simulink model "L6"  (R2019b)
settings: Solver=VariableStepAuto  StartTime=0.0  StopTime=50  RelTol=1e-3
InitFcn:
  | %% Параметры механизма
  | m = [1 1];      % масса звеньев
  | l = [1 1];      % длина звеньев
  | lc = [.5 .5];   % расст от СК звена до центра масс звена
  | I = [1 1];      % моменты инерции звеньев
  | Jm = [0 0];     % момент инерции редукторов?
  | r = [1 1];      % передаточные числа редукторов
  | D = [.1 .1];    % агрегированные коэффициенты демпфирования
  | 
  | g = 9.81;       % ускорение свободного падения
  | 
  | 
  | global rho;
  | rho = [
  |     m(1)*lc(1)^2 + m(2)*l(1)^2 + 2*m(2)*l(1)*lc(2)^2 + I(1),... % rho_1
  |     m(2)*lc(2)^2 + I(2),...                                     % rho_2
  |     m(2)*l(1)*lc(2),...                                         % rho_3
  |     r(1)^2*Jm(1),...                                            % rho_4
  |     r(2)^2*Jm(2),...                                            % rho_5
  |     (m(1)*lc(1) + m(2)*l(1))*g,...                              % rho_6
  |     m(2)*lc(2)*g,...                                            % rho_7
  |     m(2)*lc(2),...                                              % rho_8
  |     r(1)^2*D(1),...                                             % rho_9
  |     r(2)^2*D(2)                                                 % rho_10
  |     ];
  | 
  | 
  | q_ref = [1 2];
  | c2 = cos(q_ref(2));
  | 
  | % матрица номинального момента инерции манипулятора
  | M0 = [
  |     rho(1) + rho(2) + 2*rho(3)*c2 + rho(4), rho(2) + rho(3)*c2;
  |     rho(2) + rho(3)*c2, rho(2) + rho(5);
  |     ];
  | 
  | % матрица вязкого трения
  | Friction = [
  |     rho(9) 0;
  |     0 rho(10)
  |     ];
  | 
  | %% Параметры генераторов
  | % Задающий блок
  | A_ref = [1 1];      % амплитуды
  | psi_ref = [0 0];    % фазы
  | omega_ref = [1 2];  % частоты
  | 
  | w_ref_0 = [
  |     A_ref(1)*sin(psi_ref(1)),...
  |     omega_ref(1)*A_ref(1)*cos(psi_ref(1)),...
  |     A_ref(2)*sin(psi_ref(2)),...
  |     omega_ref(2)*A_ref(2)*cos(psi_ref(2))
  |     ]';
  | 
  | Sref1 = [
  |     0 1;
  |     -omega_ref(1)^2 0
  |     ];
  | Sref2 = [
  |     0 1;
  |     -omega_ref(2)^2 0
  |     ];
  | 
  | Sref = blkdiag(Sref1, Sref2);
  | 
  | H_ref_p1 = [1 0];
  | H_ref_p2 = [1 0];
  | H_ref_p = blkdiag(H_ref_p1, H_ref_p2);
  | 
  | H_ref_v1 = [0 1];
  | H_ref_v2 = [0 1];
  | H_ref_v = blkdiag(H_ref_v1, H_ref_v2);
  | 
  | H_ref_a1 = [-omega_ref(1)^2 0];
  | H_ref_a2 = [-omega_ref(2)^2 0];
  | H_ref_a = blkdiag(H_ref_a1, H_ref_a2);
  | 
  | % Возмущающий блок
  | A_dist = [30 40];       % амплитуды
  | C_dist = [5 6];         % свободный член
  | psi_dist = [7 8];       % фазы
  | omega_dist = [1 2];     % частоты
  | 
  | w_dist_0 = [
  |     C_dist(1);
  |     A_dist(1)*sin(psi_dist(1));
  |     omega_dist(1)*A_dist(1)*cos(psi_dist(1));
  |     C_dist(2);
  |     A_dist(2)*sin(psi_dist(2));
  |     omega_dist(2)*A_dist(2)*cos(psi_dist(2))
  |     ];
  | 
  | Sdist1 = [
  |     0 0 0
  |     0 0 1;
  |     0 -omega_dist(1)^2 0
  |     ];
  | Sdist2 = [
  |     0 0 0
  |     0 0 1;
  |     0 -omega_dist(2)^2 0
  |     ];
  | 
  | Sdist = blkdiag(Sdist1, Sdist2);
  | 
  | H_dist_1 = [1 1 0];
  | H_dist_2 = [1 1 0];
  | H_dist = blkdiag(H_dist_1, H_dist_2);
  | 
  | f = [1 3 3];
  | F_1 =[
  |     zeros(2, 1) eye(2);
  |     -f
  |     ];
  | F_2 =[
  |     zeros(2, 1) eye(2);
  |     -f
  |     ];
  | F = blkdiag(F_1, F_2);
  | 
  | G_1 = [0 0 1]';
  | G_2 = [0 0 1]';
  | G = blkdiag(G_1, G_2);
  | 
  | Gamma_1 = f - [0 omega_dist(1)^2 0];
  | Gamma_2 = f - [0 omega_dist(2)^2 0];
  | Gamma = blkdiag(Gamma_1, Gamma_2);
  | %% Параметры регулятора
  | kappa = 1000;
  | 
  | K =[
  |     1 0 1 0;
  |     0 1 0 1
  |     ];
  | 
  | N = inf;
  | 
  | A0 = [
  |     30 3;
  |     3 30
  |     ];
  | A1 = [
  |     30 3;
  |     3 30
  |     ];
  | A2 = [
  |     10 1;
  |     1 10
  |     ];
  | 
  | A = [
  |     -A2 eye(size(A2)) zeros(size(A2));
  |     -A1 zeros(size(A1)) eye(size(A1));
  |     -A0 zeros(size(A0)) zeros(size(A0));
  |     ];
  | % остальные матрицы зависят от q и объявлены функциями
settings Model: Creator=bedla  LastModifiedBy=bedla

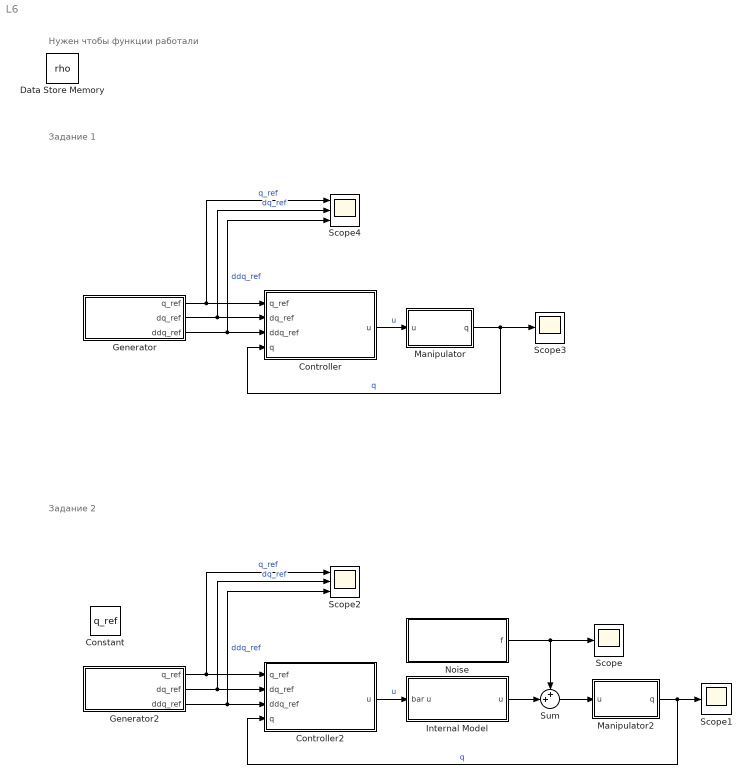
== system L6 ==
  note: Задание 1
  note: Нужен чтобы функции работали
  note: Задание 2
  Constant : Constant  Value=q_ref
  Controller : Subsystem
  Controller2 : Subsystem
  Data Store Memory : DataStoreMemory  DataStoreName=rho  ReadBeforeWriteMsg=warning  WriteAfterWriteMsg=warning  WriteAfterReadMsg=warning  InitialValue=rho  ShowAdditionalParam=off  OutDataTypeStr=double
  Generator : Subsystem
  Generator2 : Subsystem
  Internal Model : Subsystem
  Manipulator : Subsystem
  Manipulator2 : Subsystem
  Noise : Subsystem
  Scope : Scope
  Scope1 : Scope
  Scope2 : Scope  NumInputPorts=3
  Scope3 : Scope
  Scope4 : Scope  NumInputPorts=3
  Sum : Sum  Inputs=++|
  wires:
  Generator/1(q_ref) -> Controller/1(q_ref), Scope4/1  "q_ref"
  Manipulator/1(q) -> Controller/4(q), Scope3/1  "q"
  Generator/3(ddq_ref) -> Controller/3(ddq_ref), Scope4/3  "ddq_ref"
  Controller/1(u) -> Manipulator/1(u)  "u"
  Generator/2(dq_ref) -> Controller/2(dq_ref), Scope4/2  "dq_ref"
  Generator2/2(dq_ref) -> Controller2/2(dq_ref), Scope2/2  "dq_ref"
  Generator2/3(ddq_ref) -> Controller2/3(ddq_ref), Scope2/3  "ddq_ref"
  Generator2/1(q_ref) -> Scope2/1, Controller2/1(q_ref)  "q_ref"
  Controller2/1(u) -> Internal Model/1(bar u)  "u"
  Manipulator2/1(q) -> Controller2/4(q), Scope1/1  "q"
  Sum/1 -> Manipulator2/1(u)
  Noise/1(f) -> Scope/1, Sum/1
  Internal Model/1(u) -> Sum/2

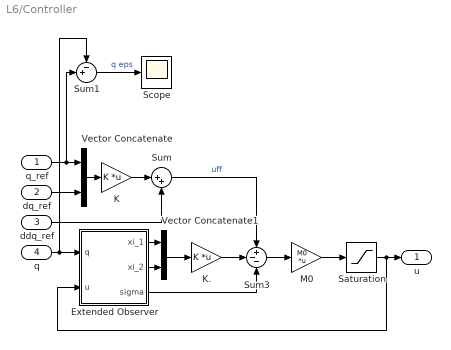
== system L6/Controller ==
  q_ref : Inport
  dq_ref : Inport  Port=2
  ddq_ref : Inport  Port=3
  q : Inport  Port=4
  Extended Observer : Subsystem
  K : Gain  Gain=K  Multiplication=Matrix(K*u) (u vector)
  K. : Gain  Gain=K  Multiplication=Matrix(K*u) (u vector)
  M0 : Gain  Gain=M0  Multiplication=Matrix(K*u) (u vector)
  Saturation : Saturate  UpperLimit=N  LowerLimit=-N
  Scope : Scope
  Sum : Sum  Inputs=|++
  Sum1 : Sum  Inputs=-+|
  Sum3 : Sum  Inputs=+--
  Vector Concatenate : Concatenate
  Vector Concatenate1 : Concatenate
  u : Outport
  wires:
  Saturation/1 -> Extended Observer/2(u), u/1
  dq_ref/1 -> Vector Concatenate/2
  q_ref/1 -> Sum1/2, Vector Concatenate/1
  Vector Concatenate/1 -> K/1
  K/1 -> Sum/1
  ddq_ref/1 -> Sum/2
  Sum3/1 -> M0/1
  Extended Observer/3(sigma) -> Sum3/3
  K./1 -> Sum3/2
  M0/1 -> Saturation/1
  Extended Observer/2(xi_2) -> Vector Concatenate1/2
  Sum/1 -> Sum3/1  "uff"
  q/1 -> Sum1/1, Extended Observer/1(q)
  Extended Observer/1(xi_1) -> Vector Concatenate1/1
  Vector Concatenate1/1 -> K./1
  Sum1/1 -> Scope/1  "q eps"

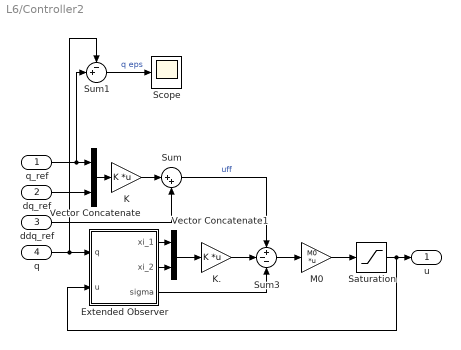
== system L6/Controller2 ==
  q_ref : Inport
  dq_ref : Inport  Port=2
  ddq_ref : Inport  Port=3
  q : Inport  Port=4
  Extended Observer : Subsystem
  K : Gain  Gain=K  Multiplication=Matrix(K*u) (u vector)
  K. : Gain  Gain=K  Multiplication=Matrix(K*u) (u vector)
  M0 : Gain  Gain=M0  Multiplication=Matrix(K*u) (u vector)
  Saturation : Saturate  UpperLimit=N  LowerLimit=-N
  Scope : Scope
  Sum : Sum  Inputs=|++
  Sum1 : Sum  Inputs=-+|
  Sum3 : Sum  Inputs=+--
  Vector Concatenate : Concatenate
  Vector Concatenate1 : Concatenate
  u : Outport
  wires:
  Saturation/1 -> Extended Observer/2(u), u/1
  dq_ref/1 -> Vector Concatenate/2
  q_ref/1 -> Sum1/2, Vector Concatenate/1
  Vector Concatenate/1 -> K/1
  K/1 -> Sum/1
  ddq_ref/1 -> Sum/2
  Sum3/1 -> M0/1
  Extended Observer/3(sigma) -> Sum3/3
  K./1 -> Sum3/2
  M0/1 -> Saturation/1
  Extended Observer/2(xi_2) -> Vector Concatenate1/2
  Sum/1 -> Sum3/1  "uff"
  q/1 -> Sum1/1, Extended Observer/1(q)
  Extended Observer/1(xi_1) -> Vector Concatenate1/1
  Vector Concatenate1/1 -> K./1
  Sum1/1 -> Scope/1  "q eps"

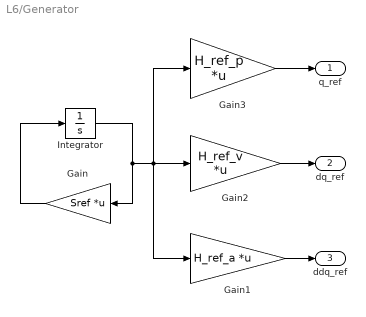
== system L6/Generator ==
  Gain : Gain  Gain=Sref  Multiplication=Matrix(K*u) (u vector)
  Gain1 : Gain  Gain=H_ref_a  Multiplication=Matrix(K*u) (u vector)
  Gain2 : Gain  Gain=H_ref_v  Multiplication=Matrix(K*u) (u vector)
  Gain3 : Gain  Gain=H_ref_p  Multiplication=Matrix(K*u) (u vector)
  Integrator : Integrator  InitialCondition=w_ref_0
  q_ref : Outport
  dq_ref : Outport  Port=2
  ddq_ref : Outport  Port=3
  wires:
  Gain/1 -> Integrator/1
  Integrator/1 -> Gain/1, Gain3/1, Gain2/1, Gain1/1
  Gain1/1 -> ddq_ref/1
  Gain2/1 -> dq_ref/1
  Gain3/1 -> q_ref/1

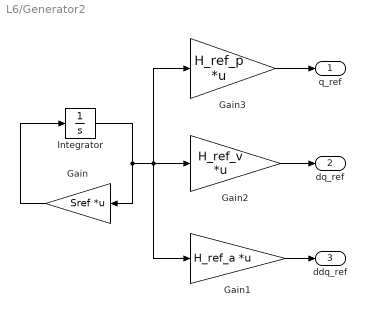
== system L6/Generator2 ==
  Gain : Gain  Gain=Sref  Multiplication=Matrix(K*u) (u vector)
  Gain1 : Gain  Gain=H_ref_a  Multiplication=Matrix(K*u) (u vector)
  Gain2 : Gain  Gain=H_ref_v  Multiplication=Matrix(K*u) (u vector)
  Gain3 : Gain  Gain=H_ref_p  Multiplication=Matrix(K*u) (u vector)
  Integrator : Integrator  InitialCondition=w_ref_0
  q_ref : Outport
  dq_ref : Outport  Port=2
  ddq_ref : Outport  Port=3
  wires:
  Gain/1 -> Integrator/1
  Integrator/1 -> Gain/1, Gain3/1, Gain2/1, Gain1/1
  Gain1/1 -> ddq_ref/1
  Gain2/1 -> dq_ref/1
  Gain3/1 -> q_ref/1

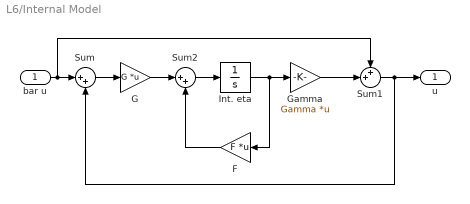
== system L6/Internal Model ==
  bar u : Inport
  F : Gain  Gain=F  Multiplication=Matrix(K*u)
  G : Gain  Gain=G  Multiplication=Matrix(K*u)
  Gamma : Gain  Gain=Gamma  Multiplication=Matrix(K*u)
  Int. eta : Integrator
  Sum : Sum  Inputs=|++
  Sum1 : Sum  Inputs=++|
  Sum2 : Sum  Inputs=|++
  u : Outport
  wires:
  bar u/1 -> Sum1/1, Sum/1
  Sum1/1 -> Sum/2, u/1
  Sum/1 -> G/1
  Gamma/1 -> Sum1/2
  Int. eta/1 -> F/1, Gamma/1
  G/1 -> Sum2/1
  Sum2/1 -> Int. eta/1
  F/1 -> Sum2/2

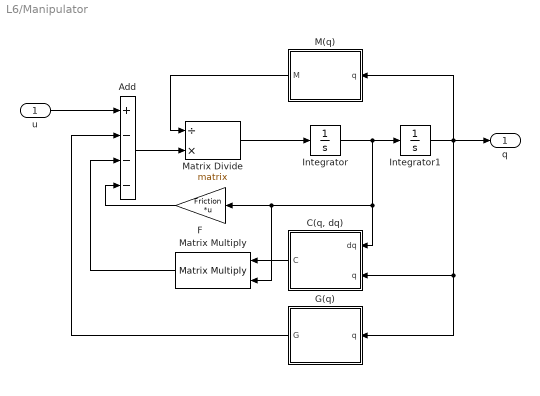
== system L6/Manipulator ==
  u : Inport
  Add : Sum  Inputs=+---
  "C(q, dq)" : MATLAB Function
  F : Gain  Gain=Friction  Multiplication=Matrix(K*u) (u vector)
  G(q) : MATLAB Function  TreatAsAtomicUnit=on
  Integrator : Integrator
  Integrator1 : Integrator
  M(q) : MATLAB Function  TreatAsAtomicUnit=on
  Matrix Divide : Product  Inputs=/*  Multiplication=Matrix(*)
  Matrix Multiply : Product  Multiplication=Matrix(*)
  q : Outport
  wires:
  Matrix Divide/1 -> Integrator/1
  Add/1 -> Matrix Divide/2
  Integrator/1 -> "C(q, dq)"/1(dq), Matrix Multiply/2, F/1, Integrator1/1
  Matrix Multiply/1 -> Add/3
  Integrator1/1 -> q/1, M(q)/1(q), G(q)/1(q), "C(q, dq)"/2(q)
  M(q)/1(M) -> Matrix Divide/1
  u/1 -> Add/1
  G(q)/1(G) -> Add/2
  "C(q, dq)"/1(C) -> Matrix Multiply/1
  F/1 -> Add/4

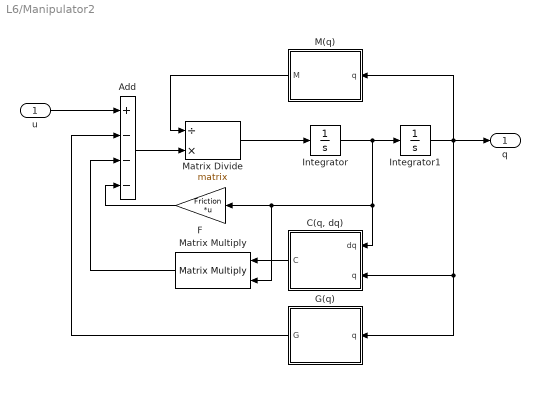
== system L6/Manipulator2 ==
  u : Inport
  Add : Sum  Inputs=+---
  "C(q, dq)" : MATLAB Function
  F : Gain  Gain=Friction  Multiplication=Matrix(K*u) (u vector)
  G(q) : MATLAB Function  TreatAsAtomicUnit=on
  Integrator : Integrator
  Integrator1 : Integrator
  M(q) : MATLAB Function  TreatAsAtomicUnit=on
  Matrix Divide : Product  Inputs=/*  Multiplication=Matrix(*)
  Matrix Multiply : Product  Multiplication=Matrix(*)
  q : Outport
  wires:
  Matrix Divide/1 -> Integrator/1
  Add/1 -> Matrix Divide/2
  Integrator/1 -> "C(q, dq)"/1(dq), Matrix Multiply/2, F/1, Integrator1/1
  Matrix Multiply/1 -> Add/3
  Integrator1/1 -> q/1, M(q)/1(q), G(q)/1(q), "C(q, dq)"/2(q)
  M(q)/1(M) -> Matrix Divide/1
  u/1 -> Add/1
  G(q)/1(G) -> Add/2
  "C(q, dq)"/1(C) -> Matrix Multiply/1
  F/1 -> Add/4

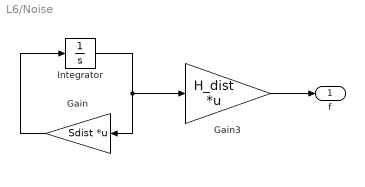
== system L6/Noise ==
  Gain : Gain  Gain=Sdist  Multiplication=Matrix(K*u) (u vector)
  Gain3 : Gain  Gain=H_dist  Multiplication=Matrix(K*u) (u vector)
  Integrator : Integrator  InitialCondition=w_dist_0
  f : Outport
  wires:
  Gain/1 -> Integrator/1
  Integrator/1 -> Gain/1, Gain3/1
  Gain3/1 -> f/1

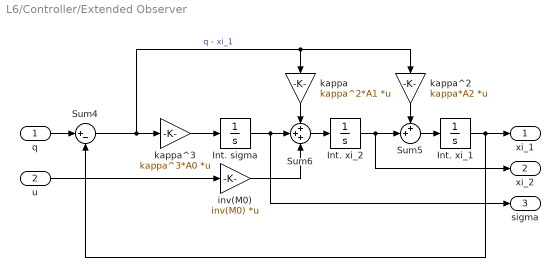
== system L6/Controller/Extended Observer ==
  q : Inport
  u : Inport  Port=2
  "Int. sigma " : Integrator
  Int. xi_1 : Integrator
  Int. xi_2 : Integrator
  Sum4 : Sum  Inputs=|+-
  Sum5 : Sum  Inputs=++|
  Sum6 : Sum  Inputs=+++
  inv(M0) : Gain  Gain=inv(M0)  Multiplication=Matrix(K*u) (u vector)
  kappa : Gain  Gain=kappa^2*A1  Multiplication=Matrix(K*u) (u vector)
  kappa^2 : Gain  Gain=kappa*A2  Multiplication=Matrix(K*u) (u vector)
  kappa^3 : Gain  Gain=kappa^3*A0  Multiplication=Matrix(K*u) (u vector)
  xi_1 : Outport
  xi_2 : Outport  Port=2
  sigma : Outport  Port=3
  wires:
  Sum6/1 -> Int. xi_2/1
  Int. xi_2/1 -> Sum5/2, xi_2/1
  "Int. sigma "/1 -> Sum6/2, sigma/1
  kappa^2/1 -> Sum5/1
  kappa/1 -> Sum6/1
  Sum4/1 -> kappa^2/1, kappa/1, kappa^3/1  "q - xi_1"
  kappa^3/1 -> "Int. sigma "/1
  inv(M0)/1 -> Sum6/3
  Sum5/1 -> Int. xi_1/1
  Int. xi_1/1 -> xi_1/1, Sum4/2
  q/1 -> Sum4/1
  u/1 -> inv(M0)/1

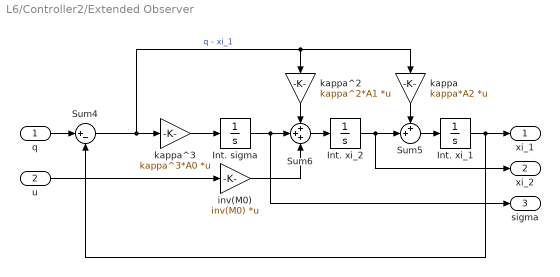
== system L6/Controller2/Extended Observer ==
  q : Inport
  u : Inport  Port=2
  "Int. sigma " : Integrator
  Int. xi_1 : Integrator
  Int. xi_2 : Integrator
  Sum4 : Sum  Inputs=|+-
  Sum5 : Sum  Inputs=++|
  Sum6 : Sum  Inputs=+++
  inv(M0) : Gain  Gain=inv(M0)  Multiplication=Matrix(K*u) (u vector)
  kappa : Gain  Gain=kappa*A2  Multiplication=Matrix(K*u) (u vector)
  kappa^2 : Gain  Gain=kappa^2*A1  Multiplication=Matrix(K*u) (u vector)
  kappa^3 : Gain  Gain=kappa^3*A0  Multiplication=Matrix(K*u) (u vector)
  xi_1 : Outport
  xi_2 : Outport  Port=2
  sigma : Outport  Port=3
  wires:
  Sum6/1 -> Int. xi_2/1
  Int. xi_2/1 -> Sum5/2, xi_2/1
  "Int. sigma "/1 -> Sum6/2, sigma/1
  kappa/1 -> Sum5/1
  kappa^2/1 -> Sum6/1
  Sum4/1 -> kappa/1, kappa^2/1, kappa^3/1  "q - xi_1"
  kappa^3/1 -> "Int. sigma "/1
  inv(M0)/1 -> Sum6/3
  Sum5/1 -> Int. xi_1/1
  Int. xi_1/1 -> xi_1/1, Sum4/2
  q/1 -> Sum4/1
  u/1 -> inv(M0)/1

== matlab function L6/Manipulator2/C(q, dq) ==
  settings: updateMethod=DISCRETE
  data: dq input; q input; C output; rho data_store_memory
function C = coreolis(dq, q)
    global rho;
    s2 = sin(q(2));
    C = [
        -rho(3)*s2*dq(2) -rho(3)*s2*(dq(1) + dq(2));
        rho(3)*s2*dq(1) 0
        ];
end

== matlab function L6/Manipulator2/G(q) ==
  settings: updateMethod=DISCRETE
  data: q input; G output; rho data_store_memory
function G = gravit(q)
    global rho;
    c1 = cos(q(1));
    c12 = cos(q(1) + q(2));
    G = [
        rho(6)*c1 + rho(7)*c12;
        rho(8)*c12
        ];
end

== matlab function L6/Manipulator2/M(q) ==
  settings: updateMethod=DISCRETE
  data: q input; M output; rho data_store_memory
function M = moments(q)
    global rho;
    c2 = cos(q(2));
    M = [
        rho(1) + rho(2) + 2*rho(3)*c2 + rho(4), rho(2) + rho(3)*c2;
        rho(2) + rho(3)*c2, rho(2) + rho(5);
        ];
end

== matlab function L6/Manipulator/C(q, dq) ==
  settings: updateMethod=DISCRETE
  data: dq input; q input; C output; rho data_store_memory
function C = coreolis(dq, q)
    global rho;
    s2 = sin(q(2));
    C = [
        -rho(3)*s2*dq(2) -rho(3)*s2*(dq(1) + dq(2));
        rho(3)*s2*dq(1) 0
        ];
end

== matlab function L6/Manipulator/G(q) ==
  settings: updateMethod=DISCRETE
  data: q input; G output; rho data_store_memory
function G = gravit(q)
    global rho;
    c1 = cos(q(1));
    c12 = cos(q(1) + q(2));
    G = [
        rho(6)*c1 + rho(7)*c12;
        rho(8)*c12
        ];
end

== matlab function L6/Manipulator/M(q) ==
  settings: updateMethod=DISCRETE
  data: q input; M output; rho data_store_memory
function M = moments(q)
    global rho;
    c2 = cos(q(2));
    M = [
        rho(1) + rho(2) + 2*rho(3)*c2 + rho(4), rho(2) + rho(3)*c2;
        rho(2) + rho(3)*c2, rho(2) + rho(5);
        ];
end
